simulink model "testemplanner_cs_old"  (R2020a)
settings: Solver=ode5  StartTime=0.0  StopTime=120  FixedStep=1/1000  RelTol=1e-3
PreLoadFcn:
  | mbxruntime.callbacks.PreLoadFcn(bdroot);
PostLoadFcn:
  | mbxruntime.callbacks.PostLoadFcn(bdroot);
InitFcn:
  | mbxruntime.callbacks.InitFcn(bdroot);
StartFcn:
  | mbxruntime.callbacks.StartFcn(bdroot);
StopFcn:
  | mbxruntime.callbacks.StopFcn(bdroot);
model workspace (MAT data in the model file):
  mbox_table : object (value not decoded)
  model_closed = 0
  sim_status = 0
values from neighbouring files (symbols this model uses):
  c_factor = 43.75    [emplanner_init.m]
  cf = -175016    [emplanner_init.m]
  cr = -130634    [emplanner_init.m]
  global_path_x = [0.057304 1.05668625507 2.05480936558 3.05165624935 4.04722112279 5.04150235808 6.03449985569 7.02621407764 8.01664569183 9.00579544113 9.99366409523 10.9802524329 ... (3001 elements, 3001x1)]    [global_path.mat]
  global_path_y = [8.29 8.29 8.29 8.29 8.29 8.29 8.29 8.29 8.29 8.29 8.29 8.29 ... (3001 elements, 3001x1)]    [global_path.mat]
  KD_PID_distance = 0.0    (= 0)    [emplanner_init.m]
  KD_PID_speed = 0    [emplanner_init.m]
  KI_PID_distance = 0.0    (= 0)    [emplanner_init.m]
  KI_PID_speed = 0    [emplanner_init.m]
  KP_PID_distance = 0.5    [emplanner_init.m]
  KP_PID_speed = 1.8    [emplanner_init.m]
  la = 1.265    [emplanner_init.m]
  lb = 2.947-1.265    (= 1.682)    [emplanner_init.m]
  LQR_K1 = k(:,1)'    [emplanner_init.m]
  LQR_K2 = k(:,2)'    [emplanner_init.m]
  LQR_K3 = k(:,3)'    [emplanner_init.m]
  LQR_K4 = k(:,4)'    [emplanner_init.m]
  m = 2020    [emplanner_init.m]
  rack_displacement = [-39.14 , -37.2 , -35.29 , -33.43 , -31.6 , -29.81 , -28.06 , -26.34 , -24.66 ,      -23.01 , -21.38 , -19.79 , -18.23 , -16.69 , -15.18 , -13.7 , -12.23 , -10.8 , -9.38 , -7.98 ,     -6.61 , -5.25 , -3.91 , -2.59 , -1.29 , 0 , 1.27 , 2.54 , 3.78 , 5.02 , 6.24 , 7.46 , 8.66 ,      9.86 , 11.05 , 12.24 , 13.41 , 14.59 , 15.76 , 16.92 , 18.09 , 19.25 , 20.42 , 21.59 , 22.76 ,      23.93 , 25.11 , 26 ...(+26 chars)    [emplanner_init.m]
  right_wheel_ground = [-70 ,-67.2 , -64.4 , -61.6 , -58.8 , -56 , -53.2 , -50.4 , -47.6 , -44.8 , -42 ,      -39.2 , -36.4 , -33.6 , -30.8 , -28 , -25.2 , -22.4 , -19.6 , -16.8 , -14 , -11.2 , -8.4 , -5.6 ,      -2.8 , 0 , 2.8 , 5.6 , 8.4 , 11.2 , 14 , 16.8 , 19.6 , 22.4 , 25.2 , 28 , 30.8 , 33.6 , 36.4 ,      39.2 , 42 , 44.8 , 47.6 , 50.4 , 53.2 , 56 , 58.8 , 61.6 , 64.4 , 67.2 , 70 ]    [emplanner_init.m]
  vx_break_point = zeros(1,5000)    [emplanner_init.m]
undefined symbols (not defined in the file or in its folder): aubr, DiscIntNeverNeededParam, tablebr, vubr
libraries: PreScanSimulinkLibrary x9, Solver_SF x1, simulink_extras x1
(part 6 of 6)

== matlab function testemplanner_cs_old/Audi_A8_Sedan_1/decision&planning module/EM_planner/Index to s ==
  data: path_x input; index2s output; path_y input; origin_point_x input; origin_point_y input; origin_match_point_index input
function index2s = fcn(path_x,path_y,origin_point_x,origin_point_y,origin_match_point_index)
    
%作用：求出frenet坐标系下的点在世界坐标系下通过index所对应的s值，即index2s
%输入：参考线、frenet坐标原点的坐标，frenet坐标原点所对应的匹配点的index
%输出：index2s：index和s之间的对应关系

%首先定义index2s数组
n=181;
index2s=zeros(181,1);

%首先计算以path起点为原点的index2s值
for i=2:n
    index2s(i)=sqrt((path_x(i)-path_x(i-1))^2+(path_y(i)-path_y(i-1))^2)+index2s(i-1);
end

%再计算从path起点到匹配点的距离S0，用上面计算的index2s减去S0即可得出真实的index2s
%s_temp =  index2s(origin_match_point_index);
%调用函数，计算路径起点的index所对应的弧长s
s = CalcSfromIndex(path_x,path_y,origin_point_x,origin_point_y,origin_match_point_index,index2s);  
%用当前点到坐标原点的s减去路径起点到坐标原点的S，就是最终的距离路径起点的s
index2s=index2s-s*ones(n,1);
end
 function s=CalcSfromIndex(ref_path_x,ref_path_y,match_point_x,match_point_y,match_point_index,index2s)   %使用一个函数来计算index所对应的S值
%%首先判断原点是在匹配点前还是匹配点后，通过向量的内积来进行判断
s_temp =  index2s(match_point_index);
vector1=[match_point_x-ref_path_x(match_point_index);match_point_y-ref_path_y(match_point_index)];
%考虑匹配点在路径终点的情况，不在终点就是匹配点和下一个点作为方向向量，如果是终点则使用匹配点和上一个点作为方向向量
if match_point_index<length(ref_path_x)
    vector2=[ref_path_x(match_point_index+1)-ref_path_x(match_point_index);ref_path_y(match_point_index+1)-ref_path_y(match_point_index)];
else
     vector2=[ref_path_x(match_point_index)-ref_path_x(match_point_index-1);ref_path_y(match_point_index)-ref_path_y(match_point_index-1)];
end
result=vector1'*vector2;    
if result >0 %原点在匹配点后，加上这个距离
    s=s_temp+sqrt(vector1'*vector1);
else        %原点在匹配点前，减去这个距离
    s=s_temp-sqrt(vector1'*vector1);
end
end

== matlab function testemplanner_cs_old/Audi_A8_Sedan_1/decision&planning module/EM_planner/general fast algorithm to find projection point info1 ==
  data: x_set input; match_point_index_set output; y_set input; path_x input; path_y input; proj_x_set output; proj_y_set output; proj_heading_set output; proj_kappa_set output; path_heading input; path_kappa input
function [match_point_index_set,proj_x_set,proj_y_set,proj_heading_set,proj_kappa_set] = fcn(x_set,y_set,path_x,path_y,path_heading,path_kappa)
%该函数是一个通用函数，找到x_set,y_set在path_x,path_y的匹配点的编号，以及投影点在直角坐标系下的(x,y,theta,kappa)
%最多可以处理128个点

match_point_index_set = ones(128,1)*nan;
proj_x_set = ones(128,1)*nan;
proj_y_set = ones(128,1)*nan;
proj_heading_set = ones(128,1)*nan;
proj_kappa_set = ones(128,1)*nan;

persistent is_first_run;
persistent init_search_index_set;
persistent pre_frenet_path_x;
persistent pre_frenet_path_y;
persistent pre_frenet_path_heading;
persistent pre_frenet_path_kappa;
if isempty(is_first_run)
    is_first_run = 0; 
    init_search_index_set = ones(128,1)*nan;
    start_index = 1;
    pre_frenet_path_x = path_x;
    pre_frenet_path_y = path_y;
    pre_frenet_path_heading = path_heading;
    pre_frenet_path_kappa = path_kappa;
    for i = 1:length(x_set)
        if isnan(x_set(i))
            break;
        else
            increase_count = 0;
            min_distance = 1e10;
            for j = start_index:length(path_x)
                distance = (x_set(i)-path_x(j))^2 + (y_set(i)-path_y(j))^2;
                if (min_distance > distance)
                    min_distance = distance;
                    init_search_index_set(i)=j;
                    increase_count = 0;
                else
                    increase_count = increase_count + 1;
                end
                if increase_count > 50
                    break;
                end
            end
            match_point_index = init_search_index_set(i);
            match_point_index_set(i) = match_point_index;
            vector_match_point = [path_x(match_point_index);path_y(match_point_index)];
            vector_match_point_direction = [cos(path_heading(match_point_index));sin(path_heading(match_point_index))];
            vector_host_point = [x_set(i);y_set(i)];
            vector_d = vector_host_point - vector_match_point;
            vector_err = (vector_d'* vector_match_point_direction) * vector_match_point_direction;
            vector_proj = vector_err + vector_match_point;
            proj_x_set(i) = vector_proj(1);
            proj_y_set(i) = vector_proj(2);
            proj_heading_set(i) = path_heading(match_point_index) + path_kappa(match_point_index) * (vector_d'* vector_match_point_direction);
            proj_kappa_set(i) = path_kappa(match_point_index);            
        end
    end 
    init_search_index_set=match_point_index_set;
else
    min_distance = inf;
    for i = 1:length(x_set)
        increase_count = 0;
        count_limit=5;
        if isnan(init_search_index_set(i))
            start_index = 1;
            count_limit=50;
       
        
        else
            
            start_index = init_search_index_set(i);
          
         end  
            
            vector_m_init = [pre_frenet_path_x(start_index);pre_frenet_path_y(start_index)];
            vector_direction_init = [cos(pre_frenet_path_heading(start_index));sin(pre_frenet_path_heading(start_index))];
            ds = vector_m_init'*vector_direction_init;
            if ds > 0.001            
                for j = start_index:length(pre_frenet_path_x )
                    distance = (x_set(i)-pre_frenet_path_x (j))^2 + (y_set(i)-pre_frenet_path_y(j))^2;
                    if (min_distance > distance)
                        min_distance = distance;
                        init_search_index_set(i)=j;
                        increase_count = 0;
                    else
                        increase_count = increase_count + 1;
                    end
                    if increase_count > count_limit
                        break;
                    end
                end
            elseif ds < -0.001
                for j = start_index:-1:1
                    distance = (x_set(i)-pre_frenet_path_x (j))^2 + (y_set(i)-pre_frenet_path_y(j))^2;
                    if (min_distance > distance)
                        min_distance = distance;
                        init_search_index_set(i)=j;
                        increase_count = 0;
                    else
                        increase_count = increase_count + 1;
                    end
                    if increase_count >  count_limit
                        break;
                    end
                end
            end
            match_point_index = init_search_index_set(i);
            match_point_index_set(i) = match_point_index;
            vector_match_point = [pre_frenet_path_x(match_point_index);pre_frenet_path_y(match_point_index)];
            vector_match_point_direction = [cos(pre_frenet_path_heading(match_point_index));sin(pre_frenet_path_heading(match_point_index))];
            vector_host_point = [x_set(i);y_set(i)];
            vector_d = vector_host_point - vector_match_point;
            vector_err = (vector_d'* vector_match_point_direction) * vector_match_point_direction;
            vector_proj = vector_err + vector_match_point;
            proj_x_set(i) = vector_proj(1);
            proj_y_set(i) = vector_proj(2);
            proj_heading_set(i) = pre_frenet_path_heading(match_point_index) + pre_frenet_path_kappa(match_point_index) * (vector_d'* vector_match_point_direction);
            proj_kappa_set(i) = pre_frenet_path_kappa(match_point_index);            
        end
    end    
    init_search_index_set = match_point_index_set;
    pre_frenet_path_x = path_x;
    pre_frenet_path_y = path_y;
    pre_frenet_path_heading = path_heading;
    pre_frenet_path_kappa = path_kappa;
end
